simulink model "vehicle_model_2025"  (R2025a)
settings: Solver=ode23tb  StartTime=0.0  StopTime=20  MaxStep=0.001  RelTol=1e-3
model workspace (MAT data in the model file):
  init_r = 0
  init_vx = 0
  init_vy = 0
values from neighbouring files (symbols this model uses):
  Par =     [0_Load_data.mat]
  TireData =     [0_Load_data.mat]
undefined symbols (not defined in the file or in its folder): aero_par, Battery, Motor, SimInput_Steer, SimInput_TorqueFL, SimInput_TorqueFR, SimInput_TorqueRL, SimInput_TorqueRR, sus_par
libraries: simulink x4, BatteryEstimators x1
(part 1 of 2)
settings Model: PauseTimes=0  PacingRate=0.001000  Creator=rajde  LastModifiedBy=vishal bhujbal
settings DataIOCC: SaveOutput=off  SaveTime=off
settings DebuggingCC: UnderSpecifiedDimensionMsg=warning

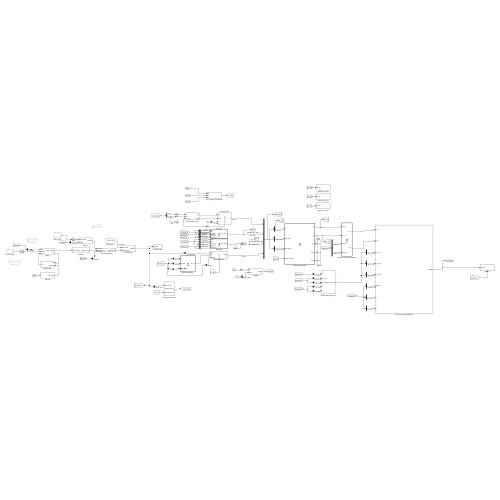
[thumbnail: Simulink's stored preview of the top-level diagram]
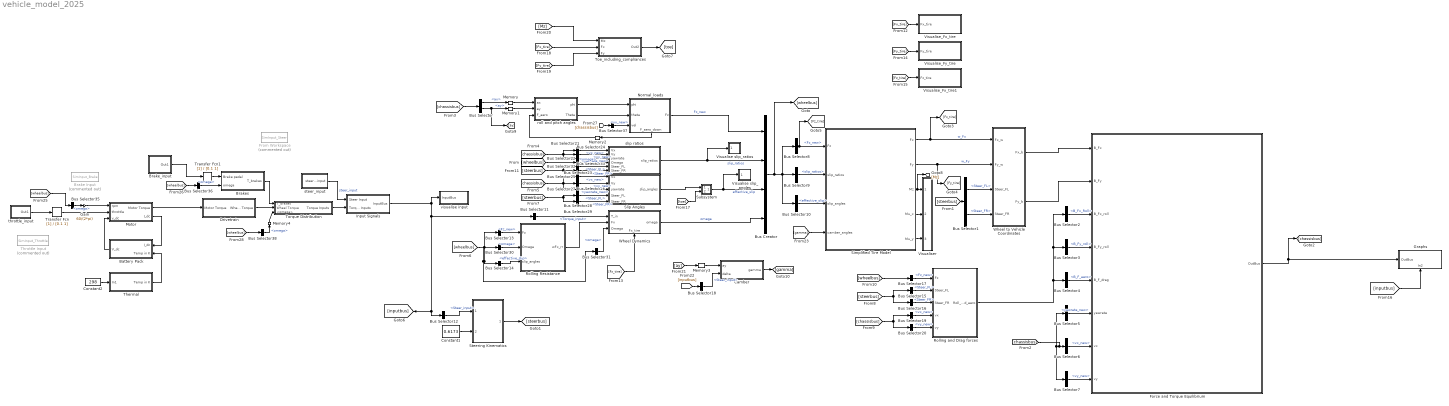
== system vehicle_model_2025 ==
  Battery Pack : Subsystem
  Brake Input : FromWorkspace  Commented=on  VariableName=SimInput_Brake
  Brake_input : Subsystem
  Brakes : Subsystem
  Bus Creator : BusCreator  Inputs=4
  Bus Selector : BusSelector  OutputSignals=ax,ay
  Bus Selector1 : BusSelector  OutputSignals=Steer_FL,Steer_FR
  Bus Selector10 : BusSelector  OutputSignals=effective_slip
  Bus Selector11 : BusSelector  OutputSignals=Torque_input
  Bus Selector12 : BusSelector  OutputSignals=Steer_input
  Bus Selector13 : BusSelector  OutputSignals=Fz_new
  Bus Selector14 : BusSelector  OutputSignals=effective_slip
  Bus Selector15 : BusSelector  OutputSignals=Steer_FL
  Bus Selector16 : BusSelector  OutputSignals=Steer_FR
  Bus Selector17 : BusSelector  OutputSignals=Fz_new
  Bus Selector18 : BusSelector  OutputSignals=Steer_input
  Bus Selector{6,19,21,25,37} (5 alike) : BusSelector  OutputSignals=vx_new
  Bus Selector2 : BusSelector  OutputSignals=B_Fx_Roll
  Bus Selector{7,20,24,26} (4 alike) : BusSelector  OutputSignals=vy_new
  Bus Selector22 : BusSelector  OutputSignals=yawrate_new
  Bus Selector{23,30..31,35..36,38} (6 alike) : BusSelector  OutputSignals=omega
  Bus Selector27 : BusSelector  OutputSignals=yawrate_new
  Bus Selector28 : BusSelector  OutputSignals=Steer_FL
  Bus Selector29 : BusSelector  OutputSignals=Steer_FR
  Bus Selector3 : BusSelector  OutputSignals=B_Fy_roll
  Bus Selector32 : BusSelector  OutputSignals=Steer_FL
  Bus Selector33 : BusSelector  OutputSignals=Steer_FR
  Bus Selector4 : BusSelector  OutputSignals=B_F_aero
  Bus Selector5 : BusSelector  OutputSignals=yawrate_new
  Bus Selector8 : BusSelector  OutputSignals=Fz_new
  Bus Selector9 : BusSelector  OutputSignals=slip_ratios
  Camber : Subsystem
  Constant1 : Constant  Value=0.6173
  Constant2 : Constant  Value=298
  Drivetrain : Subsystem
  Force and Torque Equilibrium : Subsystem
  From Workspace : FromWorkspace  Commented=on  VariableName=SimInput_Steer
  Gain : Gain  Gain=60/(2*pi)
  Graphs : Subsystem
      settings: PortSchema="{\"entries\":[{\"content\":{\"sides\":[{\"content\":{\"connectorIds\":[\"In1\"]},\"type\":\"ConnectorPlacement.EquallySpacedRectSide\",\"uuid\":\"0d7f1a6c-503e-4c9f-90e9-70f717dd7dfc\"},{\"content\":{\"side\":\"RIGHT\"},\"type\":\"ConnectorPlacement.EquallySpacedRectSide\",\"uuid\":\"62097468-b066-4e29-8f99-7427d14bee77\"},{\"content\":{\"side\":\"TOP\"},\"type\":\"ConnectorPlacement.EquallySpacedRectSide\",\"uuid\":\"2a3f381e-a201-4804-99b7-77b73504b102\"},{\"content\":{\"connectorIds\":[\"In2\"],\"side\":\"BOTTOM\"},\"type\":\"ConnectorPlacement.EquallySpacedRectSide\",\"uuid\":\"dae5de0a-879c-4844-a347-7056417d054f\"}]},\"type\":\"ConnectorPlacement.EquallySpacedConnector\",\"uuid\":\"aa2835d0-6748-4566-adf9-84e8214dd5a8\"}],\"packageUris\":[\"http://schema.mathworks.com/mf0/Connector/R2020b\"],\"version\":\"1.0\"}"
  Input Signals : Subsystem
  Memory : Memory  InheritSampleTime=on
  Memory1 : Memory  InheritSampleTime=on
  Memory2 : Memory  InheritSampleTime=on
  Memory3 : Memory
  Memory4 : Memory
  Motor : Subsystem
  Normal_loads : Subsystem
      settings: PortSchema="{\"entries\":[{\"content\":{\"sides\":[{\"content\":{\"connectorIds\":[\"In1\",\"In2\",\"In3\"]},\"type\":\"ConnectorPlacement.EquallySpacedRectSide\",\"uuid\":\"5b7db607-33bd-4d54-b958-3aa960e46147\"},{\"content\":{\"connectorIds\":[\"Out1\"],\"side\":\"RIGHT\"},\"type\":\"ConnectorPlacement.EquallySpacedRectSide\",\"uuid\":\"c12df481-c511-4c4c-afb1-8a5812ce44a5\"},{\"content\":{\"side\":\"TOP\"},\"type\":\"ConnectorPlacement.EquallySpacedRectSide\",\"uuid\":\"2c6024fe-fe45-4ba9-a61f-594b86562523\"},{\"content\":{\"connectorIds\":[\"Out2\"],\"side\":\"BOTTOM\"},\"type\":\"ConnectorPlacement.EquallySpacedRectSide\",\"uuid\":\"099189a9-186d-4ac0-a0af-1ec3a070ea03\"}]},\"type\":\"ConnectorPlacement.EquallySpacedConnector\",\"uuid\":\"81c2e338-68e5-401a-bb4f-0a973fbf41e6\"}],\"packageUris\":[\"http://schema.mathworks.com/mf0/Connector/R2020b\"],\"version\":\"1.0\"}"
  Rolling Resistance : MATLAB Function  TreatAsAtomicUnit=on
  Rolling and Drag forces : Subsystem
  Simplified Tire Model : MATLAB Function  TreatAsAtomicUnit=on
  Slip Angles : MATLAB Function  TreatAsAtomicUnit=on
  Steering Kinematics : Subsystem
  Subsystem : Subsystem
  Thermal : Subsystem
  Throttle Input : FromWorkspace  Commented=on  VariableName=SimInput_Throttle
  Toe_including_compliances : Subsystem
  Torque Distribution : Subsystem
  Transfer Fcn : TransferFcn  Denominator=[0.1 1]
  Transfer Fcn1 : TransferFcn  Denominator=[0.1 1]
  Visualise slip_angles : Subsystem
  Visualise slip_ratios : Subsystem
  Visualise_Fx_tire : Subsystem
  Visualise_Fx_tire1 : Subsystem
  Visualise_Fy_tire : Subsystem
  Visualiser : Subsystem
  Wheel Dynamics : Subsystem
      settings: PortSchema="{\"entries\":[{\"content\":{\"sides\":[{\"content\":{\"connectorIds\":[\"In1\",\"In2\",\"In3\"]},\"type\":\"ConnectorPlacement.EquallySpacedRectSide\",\"uuid\":\"f2e918e6-c6f6-4ec9-89f3-e2543a6374fd\"},{\"content\":{\"connectorIds\":[\"Out1\"],\"side\":\"RIGHT\"},\"type\":\"ConnectorPlacement.EquallySpacedRectSide\",\"uuid\":\"be700f5f-5cf3-4eec-a6f7-872bb7cd40f6\"},{\"content\":{\"side\":\"TOP\"},\"type\":\"ConnectorPlacement.EquallySpacedRectSide\",\"uuid\":\"c4f49273-9888-4d11-a98e-35dc6f585916\"},{\"content\":{\"connectorIds\":[\"In4\"],\"side\":\"BOTTOM\"},\"type\":\"ConnectorPlacement.EquallySpacedRectSide\",\"uuid\":\"8d2e7982-4362-4abb-b8fe-c155beeed1bc\"}]},\"type\":\"ConnectorPlacement.EquallySpacedConnector\",\"uuid\":\"4d6dafa1-905e-4e38-a48b-73a98e690073\"}],\"packageUris\":[\"http://schema.mathworks.com/mf0/Connector/R2020b\"],\"version\":\"1.0\"}"
  Wheel to Vehicle Coordinates : MATLAB Function  TreatAsAtomicUnit=on
  roll and pitch angles : Subsystem
  slip ratios : MATLAB Function  TreatAsAtomicUnit=on
  steer_input : Subsystem
  throttle_input : Subsystem
  visualise input : Subsystem
  wires:
  Simplified Tire Model/3(Mz) -> [Mz], Visualiser/1(mz)
  Simplified Tire Model/4(Mu_x) -> Visualiser/2(mu_x)
  Simplified Tire Model/5(Mu_y) -> Visualiser/3(mu_y)
  Simplified Tire Model/2(Fy) -> Wheel to Vehicle Coordinates/2(Fy_w), [Fy_tire]  "w_Fy"
  Simplified Tire Model/1(Fx) -> Wheel to Vehicle Coordinates/1(Fx_w), [Fx_tire]  "w_Fx"
  Wheel to Vehicle Coordinates/2(Fy_b) -> Force and Torque Equilibrium/2(B_Fy)
  Wheel to Vehicle Coordinates/1(Fx_b) -> Force and Torque Equilibrium/1(B_Fx)
  slip ratios/1(slip_ratios) -> Visualise slip_ratios/1(Kappa), Bus Creator/2  "slip_ratios"
  Wheel Dynamics/1(omega) -> Bus Creator/4  "omega"
  Bus Selector/1 -> Memory/1  "<ax>"
  Rolling Resistance/1(wFx_rr) -> Wheel Dynamics/2(Fx)
  Bus Selector1/1 -> Wheel to Vehicle Coordinates/3(Steer_FL)  "<Steer_FL>"
  Bus Selector1/2 -> Wheel to Vehicle Coordinates/4(Steer_FR)  "<Steer_FR>"
  Rolling and Drag forces/1(Roll_and_aero) -> Bus Selector2/1, Bus Selector3/1, Bus Selector4/1
  Bus Selector2/1 -> Force and Torque Equilibrium/3(B_Fx_roll)  "<B_Fx_Roll>"
  Bus Selector3/1 -> Force and Torque Equilibrium/4(B_Fy_roll)  "<B_Fy_roll>"
  Bus Selector4/1 -> Force and Torque Equilibrium/5(B_F_drag)  "<B_F_aero>"
  Bus Selector5/1 -> Force and Torque Equilibrium/6(yawrate)  "<yawrate_new>"
  Force and Torque Equilibrium/1(OutBus) -> [chassisbus], Graphs/1(OutBus)
  Bus Selector7/1 -> Force and Torque Equilibrium/8(vy)  "<vy_new>"
  Bus Selector6/1 -> Force and Torque Equilibrium/7(vx)  "<vx_new>"
  Bus Selector8/1 -> [Fz_tire], Simplified Tire Model/1(Fz)  "<Fz_new>"
  Bus Selector10/1 -> Simplified Tire Model/3(slip_angles)  "<effective_slip>"
  Bus Selector9/1 -> Simplified Tire Model/2(slip_ratios)  "<slip_ratios>"
  Bus Creator/1 -> [wheelbus], Bus Selector10/1, Bus Selector8/1, Bus Selector9/1
  Bus Selector12/1 -> Steering Kinematics/1(Steer_Input)  "<Steer_input>"
  Bus Selector11/1 -> Wheel Dynamics/1(T_in)  "<Torque_input>"
  Input Signals/1(InputBus) -> visualise input/1(InputBus), Bus Selector12/1, [inputbus], Bus Selector11/1
  Bus Selector14/1 -> Rolling Resistance/3(slip_angles)  "<effective_slip>"
  Bus Selector15/1 -> Rolling and Drag forces/2(Steer_FL)  "<Steer_FL>"
  Bus Selector16/1 -> Rolling and Drag forces/3(Steer_FR)  "<Steer_FR>"
  Constant1/1 -> Steering Kinematics/2(Ackermann_Pct)
  Bus Selector17/1 -> Rolling and Drag forces/1(Fz)  "<Fz_new>"
  Bus Selector19/1 -> Rolling and Drag forces/4(vx)  "<vx_new>"
  Bus Selector20/1 -> Rolling and Drag forces/5(vy)  "<vy_new>"
  Bus Selector21/1 -> slip ratios/1(Vx)  "<vx_new>"
  Bus Selector22/1 -> slip ratios/3(yawrate)  "<yawrate_new>"
  Bus Selector23/1 -> slip ratios/4(Omega)  "<omega>"
  Bus Selector25/1 -> Slip Angles/1(Vx)  "<vx_new>"
  Bus Selector26/1 -> Slip Angles/2(Vy)  "<vy_new>"
  Bus Selector27/1 -> Slip Angles/3(yawrate)  "<yawrate_new>"
  Bus Selector28/1 -> Slip Angles/4(Steer_FL)  "<Steer_FL>"
  Bus Selector29/1 -> Slip Angles/5(Steer_FR)  "<Steer_FR>"
  Steering Kinematics/1(Steering Angles) -> [steerbus]
  [steerbus] -> Bus Selector1/1
  [chassisbus] -> Bus Selector5/1, Bus Selector7/1, Bus Selector6/1
  [chassisbus] -> Bus Selector/1
  Bus Selector/2 -> Memory1/1, [ay]  "<ay>"
  [wheelbus] -> Bus Selector23/1
  [chassisbus] -> Bus Selector22/1, Bus Selector24/1, Bus Selector21/1
  [chassisbus] -> Bus Selector27/1, Bus Selector26/1, Bus Selector25/1
  [steerbus] -> Bus Selector29/1, Bus Selector28/1
  [wheelbus] -> Bus Selector13/1, Bus Selector30/1, Bus Selector14/1, Bus Selector31/1
  Bus Selector30/1 -> Rolling Resistance/2(Omega)  "<omega>"
  Bus Selector31/1 -> Wheel Dynamics/3(Omega)  "<omega>"
  [steerbus] -> Bus Selector16/1, Bus Selector15/1
  [chassisbus] -> Bus Selector20/1, Bus Selector19/1
  [wheelbus] -> Bus Selector17/1
  Bus Selector24/1 -> slip ratios/2(Vy)  "<vy_new>"
  Bus Selector33/1 -> slip ratios/6(Steer_FR)  "<Steer_FR>"
  [steerbus] -> Bus Selector32/1, Bus Selector33/1
  Bus Selector32/1 -> slip ratios/5(Steer_FL)  "<Steer_FL>"
  [Fx_tire] -> Wheel Dynamics/4(Fx_tire)
  Bus Selector13/1 -> Rolling Resistance/1(Fz)  "<Fz_new>"
  [inputbus] -> Graphs/2(In2)
  Slip Angles/1(slip_angles) -> Subsystem/1(slip_angles)
  [toe] -> Subsystem/2(toe)
  Subsystem/1(Out1) -> Visualise slip_angles/1(slip_angles), Bus Creator/3  "effective_slip"
  [Mz] -> Toe_including_compliances/1(Mz)
  [Fx_tire] -> Toe_including_compliances/2(Fx)
  [Fy_tire] -> Toe_including_compliances/3(Fy)
  Toe_including_compliances/1(Out2) -> [toe]
  [ay] -> Memory3/1
  [inputbus] -> Bus Selector18/1
  Bus Selector18/1 -> Camber/2(delta)  "<Steer_input>"
  Camber/1(gamma) -> [gamma]
  [gamma] -> Simplified Tire Model/4(camber_angles)
  roll and pitch angles/2(Theta) -> Normal_loads/2(theta)
  Memory/1 -> roll and pitch angles/1(ax)
  Memory1/1 -> roll and pitch angles/2(ay)
  Memory3/1 -> Camber/1(ay)
  Memory2/1 -> roll and pitch angles/3(F_aero)
  Brakes/1(T_brakes) -> Torque Distribution/1(T_brakes)
  Motor/1(Motor Torque) -> Drivetrain/1(Motor Torque)
  Bus Selector38/1 -> Memory4/1  "<omega>"
  Bus Selector35/1 -> Gain/1  "<omega>"
  Transfer Fcn/1 -> Motor/2(throttle)
  [wheelbus] -> Bus Selector36/1
  Brake_input/1(Out1) -> Transfer Fcn1/1
  Transfer Fcn1/1 -> Brakes/1(Brake pedal)
  Drivetrain/1(Wheel Torque) -> Torque Distribution/2(Wheel Torque)
  Thermal/1(Temp in K) -> Battery Pack/2(Temp in K)
  Constant2/1 -> Thermal/1(In1)
  Gain/1 -> Motor/1(rpm)
  [wheelbus] -> Bus Selector35/1
  Motor/2(I_dc) -> Battery Pack/1(I_dc)
  Bus Selector36/1 -> Brakes/2(omega)  "<omega>"
  throttle_input/1(Out1) -> Transfer Fcn/1
  Torque Distribution/1(Torque Inputs) -> Input Signals/2(Torque Inputs)
  Battery Pack/1(V_dc) -> Motor/3(v_dc)
  [wheelbus] -> Bus Selector38/1
  steer_input/1(steer_input) -> Input Signals/1(Steer Input)  "steer_input"
  Memory4/1 -> Torque Distribution/3(<omega>)
  [Fy_tire] -> Visualise_Fy_tire/1(Fy_tire)
  [Fx_tire] -> Visualise_Fx_tire/1(Fx_tire)
  [Fz_tire] -> Visualise_Fx_tire1/1(Fz_tire)
  roll and pitch angles/1(phi) -> Normal_loads/1(phi)
  [chassisbus] -> Bus Selector37/1
  Bus Selector37/1 -> Normal_loads/3(vel)  "<vx_new>"
  Normal_loads/2(F_aero_down) -> Memory2/1
  Normal_loads/1(Fz) -> Bus Creator/1  "Fz_new"

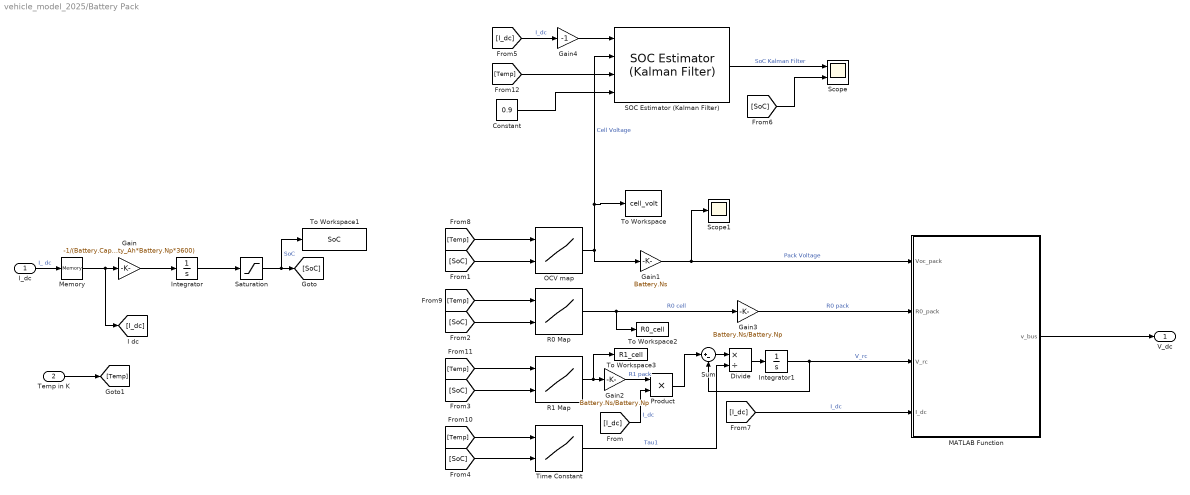
== system vehicle_model_2025/Battery Pack ==
  I_dc : Inport
  Temp in K : Inport  Port=2
  Constant : Constant  Value=0.9
  Divide : Product  Inputs=*/
  Gain : Gain  Gain=-1/(Battery.Capacity_Ah*Battery.Np*3600)
  Gain1 : Gain  Gain=Battery.Ns
  Gain2 : Gain  Gain=Battery.Ns/Battery.Np
  Gain3 : Gain  Gain=Battery.Ns/Battery.Np
  Gain4 : Gain  Gain=-1
  Integrator : Integrator  InitialCondition=1
  Integrator1 : Integrator
  MATLAB Function : MATLAB Function  TreatAsAtomicUnit=on
  Memory : Memory
  OCV map : Lookup_n-D  BreakpointsForDimension1=Battery.T_vec  BreakpointsForDimension2=Battery.SoC_vec  Table=Battery.OCV_map'  InternalRulePriority=Speed  RndMeth=Simplest
      settings: InputPortMap=u0,u1
  Product : Product
  R0 Map : Lookup_n-D  BreakpointsForDimension1=Battery.T_vec  BreakpointsForDimension2=Battery.SoC_vec  Table=Battery.R0_map'  InternalRulePriority=Speed  RndMeth=Simplest
      settings: InputPortMap=u0,u1
  R1 Map : Lookup_n-D  BreakpointsForDimension1=Battery.T_vec  BreakpointsForDimension2=Battery.SoC_vec  Table=Battery.R1_map'  InternalRulePriority=Speed  RndMeth=Simplest
      settings: InputPortMap=u0,u1
  SOC Estimator (Kalman Filter) : BatteryEstimators/SOC Estimator (Kalman Filter)  CurrentInputPartition=off  filterType=Extended Kalman filter  alpha=1  beta=2  kappa=0  Q=|  Q_2RC=|  R=0.1  P0=[1e-5 0; 0 1]  P0_2RC=[1e-5 0 0; 0 1 0;0 0 1]  Ts=1  chargeDynamics=One time-constant dynamics  SOC_vec=[0 0.1 0.25 0.5 0.75 0.9 1]  T_vec=[278 293 313]  R0_mat=[0.0117 0.0085 0.009;0.011 0.0085 0.009;0.0114 0.0087 0.0092;0.0107 0.0082 0.0088;0.0107 0.0083 0.0091;0.0113 0.0085 0.0089;0.0116 0.0085 0.0089]  R1_mat=[0.0109 0.0029 0.0013;0.0069 0.0024 0.0012;0.0047 0.0026 0.0013;0.0034 0.0016 0.001;0.0033 0.0023 0.0014;0.0033 0.0018 0.0011;0.0028 0.0017 0.0011]  tau1_mat=[20 36 39;31 45 39;109 105 61;36 29 26;59 77 67;40 33 29;25 39 33]  R2_mat=[.0109, .0029, .0013; .0069, .0024, .0012; .0047, .0026, .0013; .0034, .0016, .001; .0033, .0023, .0014; .0033, .0018, .0011; .0028, .0017, .0011]  tau2_mat=[20, 36, 39; 31, 45, 39; 109, 105, 61; 36, 29, 26; 59, 77, 67; 40, 33, 29; 25, 39, 33]  V0_mat=[3.49 3.5 3.51;3.55 3.57 3.56;3.62 3.63 3.64;3.71 3.71 3.72;3.91 3.93 3.94;4.07 4.08 4.08;4.19 4.19 4.19]  AH=4.493  DataType=Inherit: auto
      Q=|
      | [1e-6 0;
      | 0 1e-6]
      Q_2RC=|
      | [1e-6 0 0;
      | 0 1e-6 0; 0 0 1e-6]
      settings: LibrarySourceBlock=|
      | batt_sl_lib/Estimators/SOC Estimator
      | (Kalman Filter)
  Saturation : Saturate  UpperLimit=1  LowerLimit=0
  Scope : Scope  NumInputPorts=2
      settings: ActiveDisplayYMinimum=0.74077842215921907  ActiveDisplayYMaximum=0.86213619236438077  DataLoggingVariableName=ScopeData8
  Scope1 : Scope
      settings: ActiveDisplayYMinimum=583.02637249372378  ActiveDisplayYMaximum=588.01929194514184  DataLoggingVariableName=ScopeData14
  Sum : Sum  Inputs=|+-
  Time Constant : Lookup_n-D  BreakpointsForDimension1=Battery.T_vec  BreakpointsForDimension2=Battery.SoC_vec  Table=Battery.Tau_map'  InternalRulePriority=Speed  RndMeth=Simplest
      settings: InputPortMap=u0,u1
  To Workspace : ToWorkspace  VariableName=cell_volt  SaveFormat=Timeseries  SampleTime=-1
  To Workspace1 : ToWorkspace  VariableName=SoC  SaveFormat=Timeseries  SampleTime=-1
  To Workspace2 : ToWorkspace  VariableName=R0_cell  SaveFormat=Timeseries  SampleTime=-1
  To Workspace3 : ToWorkspace  VariableName=R1_cell  SaveFormat=Timeseries  SampleTime=-1
  V_dc : Outport
  wires:
  I_dc/1 -> Memory/1  "I_ dc"
  Gain/1 -> Integrator/1
  Integrator/1 -> Saturation/1
  OCV map/1 -> To Workspace/1, SOC Estimator (Kalman Filter)/2, Gain1/1  "Cell Voltage"
  Gain1/1 -> Scope1/1, MATLAB Function/1(Voc_pack)  "Pack Voltage"
  R1 Map/1 -> To Workspace3/1, Gain2/1
  R0 Map/1 -> To Workspace2/1, Gain3/1  "R0 cell"
  Gain3/1 -> MATLAB Function/2(R0_pack)  "R0 pack"
  Gain2/1 -> Product/1  "R1 pack"
  Product/1 -> Sum/1
  Integrator1/1 -> MATLAB Function/3(V_rc), Sum/2  "V_rc"
  Sum/1 -> Divide/1
  Time Constant/1 -> Divide/2  "Tau1"
  Divide/1 -> Integrator1/1
  Constant/1 -> SOC Estimator (Kalman Filter)/4
  SOC Estimator (Kalman Filter)/1 -> Scope/1  "SoC Kalman Filter"
  MATLAB Function/1(v_bus) -> V_dc/1
  [I_dc] -> Product/2  "I_dc"
  Saturation/1 -> To Workspace1/1, [SoC]  "SoC"
  [SoC] -> Time Constant/2
  [SoC] -> R1 Map/2
  [SoC] -> R0 Map/2
  [SoC] -> OCV map/2
  [I_dc] -> Gain4/1  "I_dc"
  [SoC] -> Scope/2
  [I_dc] -> MATLAB Function/4(I_dc)  "I_dc"
  Temp in K/1 -> [Temp]
  [Temp] -> OCV map/1
  [Temp] -> R0 Map/1
  [Temp] -> R1 Map/1
  [Temp] -> Time Constant/1
  [Temp] -> SOC Estimator (Kalman Filter)/3
  Memory/1 -> [I_dc], Gain/1
  Gain4/1 -> SOC Estimator (Kalman Filter)/1

== system vehicle_model_2025/Brake_input ==
  Constant4 : Constant  Value=0
  Out1 : Outport
  wires:
  Constant4/1 -> Out1/1

== system vehicle_model_2025/Brakes ==
  Brake pedal : Inport
  omega : Inport  Port=2
  MATLAB Function : MATLAB Function  TreatAsAtomicUnit=on
  T_brakes : Outport
  wires:
  MATLAB Function/1(T_brakes) -> T_brakes/1
  omega/1 -> MATLAB Function/2(omega)
  Brake pedal/1 -> MATLAB Function/1(brake_pedal)

== system vehicle_model_2025/Camber ==
  ay : Inport
  delta : Inport  Port=2
  MATLAB Function : MATLAB Function  TreatAsAtomicUnit=on
  Mux : Mux
  gamma : Outport
  wires:
  MATLAB Function/1(gamma_FR) -> Mux/1
  MATLAB Function/2(gamma_FL) -> Mux/2
  MATLAB Function/3(gamma_RL) -> Mux/3
  MATLAB Function/4(gamma_RR) -> Mux/4
  Mux/1 -> gamma/1
  ay/1 -> MATLAB Function/1(ay)
  delta/1 -> MATLAB Function/2(delta)

== system vehicle_model_2025/Drivetrain ==
  Motor Torque : Inport
  Gear Ratio : Gain  Gain=10.05
  Overall Powertrain Efficiency : Gain  Gain=0.83
  Wheel Torque : Outport
  wires:
  Motor Torque/1 -> Gear Ratio/1
  Gear Ratio/1 -> Overall Powertrain Efficiency/1
  Overall Powertrain Efficiency/1 -> Wheel Torque/1

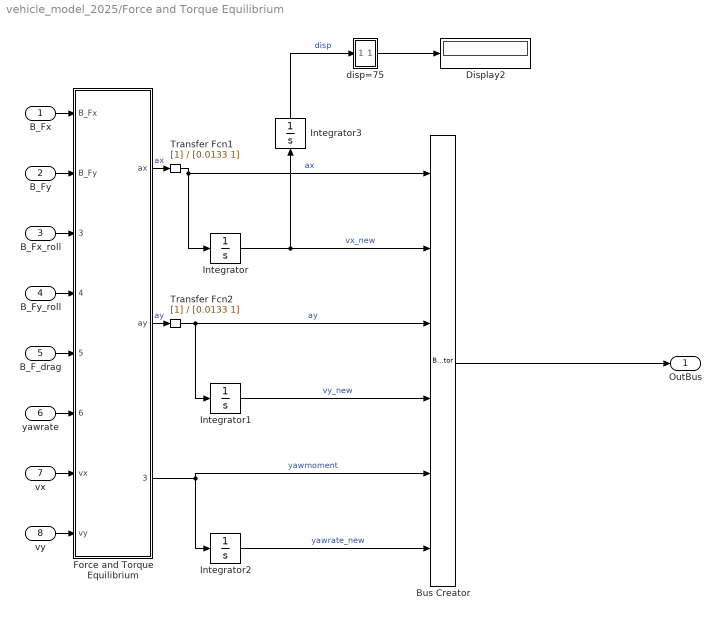
== system vehicle_model_2025/Force and Torque Equilibrium ==
  B_Fx : Inport
  B_Fy : Inport  Port=2
  B_Fx_roll : Inport  Port=3
  B_Fy_roll : Inport  Port=4
  B_F_drag : Inport  Port=5
  yawrate : Inport  Port=6
  vx : Inport  Port=7
  vy : Inport  Port=8
  Bus Creator : BusCreator  Inputs=6
  Display2 : Display
  Force and Torque Equilibrium : MATLAB Function  TreatAsAtomicUnit=on
  Integrator : Integrator  InitialCondition=init_vx  LimitOutput=on  UpperSaturationLimit=1e6  LowerSaturationLimit=0
  Integrator1 : Integrator  InitialCondition=init_vy  LimitOutput=on  UpperSaturationLimit=1e6
  Integrator2 : Integrator  InitialCondition=init_r  LimitOutput=on  UpperSaturationLimit=1e6
  Integrator3 : Integrator
  Transfer Fcn1 : TransferFcn  Denominator=[0.0133 1]
  Transfer Fcn2 : TransferFcn  Denominator=[0.0133 1]
  disp=75 : Subsystem
  OutBus : Outport
  wires:
  vy/1 -> Force and Torque Equilibrium/8(vy)
  B_Fx/1 -> Force and Torque Equilibrium/1(B_Fx)
  B_Fx_roll/1 -> Force and Torque Equilibrium/3(B_Fx_roll)
  B_F_drag/1 -> Force and Torque Equilibrium/5(B_F_drag)
  B_Fy/1 -> Force and Torque Equilibrium/2(B_Fy)
  B_Fy_roll/1 -> Force and Torque Equilibrium/4(B_Fy_roll)
  vx/1 -> Force and Torque Equilibrium/7(vx)
  Force and Torque Equilibrium/2(ay) -> Transfer Fcn2/1  "ay"
  Force and Torque Equilibrium/1(ax) -> Transfer Fcn1/1  "ax"
  Force and Torque Equilibrium/3(yawmoment) -> Integrator2/1, Bus Creator/5  "yawmoment"
  Integrator/1 -> Integrator3/1, Bus Creator/2  "vx_new"
  Integrator1/1 -> Bus Creator/4  "vy_new"
  Integrator2/1 -> Bus Creator/6  "yawrate_new"
  Bus Creator/1 -> OutBus/1
  yawrate/1 -> Force and Torque Equilibrium/6(yawrate)
  Transfer Fcn1/1 -> Integrator/1, Bus Creator/1  "ax"
  Transfer Fcn2/1 -> Integrator1/1, Bus Creator/3  "ay"
  disp=75/1(Out1) -> Display2/1
  Integrator3/1 -> disp=75/1(disp)  "disp"

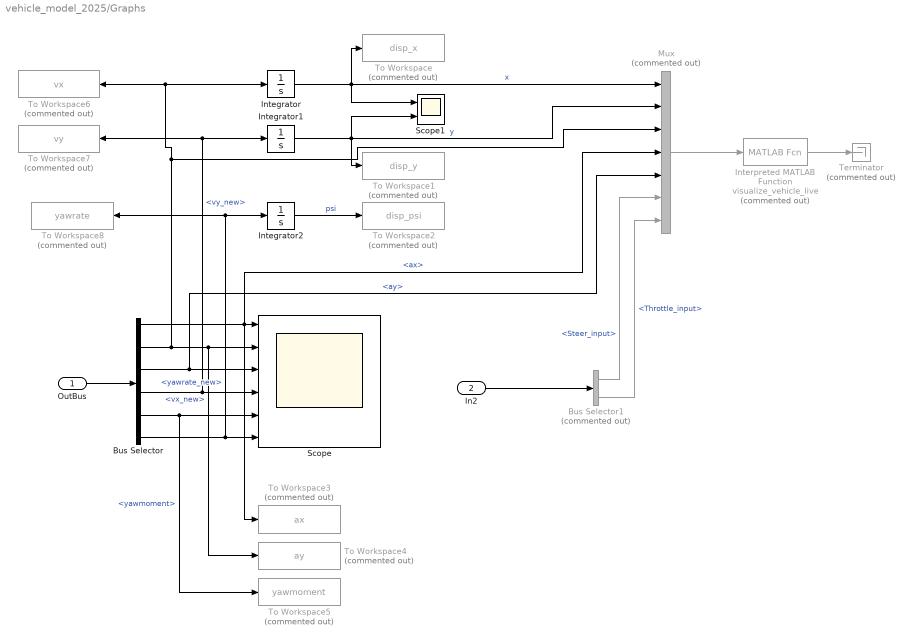
== system vehicle_model_2025/Graphs ==
  OutBus : Inport
  In2 : Inport  Port=2
  Bus Selector : BusSelector  OutputSignals=ax,vx_new,ay,vy_new,yawmoment,yawrate_new
  Bus Selector1 : BusSelector  Commented=on  OutputSignals=Steer_input,Throttle_input
  Integrator : Integrator
  Integrator1 : Integrator
  Integrator2 : Integrator
  Interpreted MATLAB Function : MATLABFcn  Commented=on  MATLABFcn=visualize_vehicle_live
  Mux : Mux  Commented=on  Inputs=7
  Scope : Scope  NumInputPorts=6
      settings: ActiveDisplayYMinimum=-0.80061135979916376  ActiveDisplayYMaximum=6.9634265458567022  DataLoggingVariableName=ScopeData2
  Scope1 : Scope  NumInputPorts=2
      settings: ActiveDisplayYMinimum=-673.27901203322881  ActiveDisplayYMaximum=6059.5111082990607  DataLoggingVariableName=ScopeData7
  Terminator : Terminator  Commented=on
  To Workspace : ToWorkspace  Commented=on  VariableName=disp_x  SaveFormat=Timeseries  SampleTime=-1
  To Workspace1 : ToWorkspace  Commented=on  VariableName=disp_y  SaveFormat=Timeseries  SampleTime=-1
  To Workspace2 : ToWorkspace  Commented=on  VariableName=disp_psi  SaveFormat=Timeseries  SampleTime=-1
  To Workspace3 : ToWorkspace  Commented=on  VariableName=ax  SaveFormat=Timeseries  SampleTime=-1
  To Workspace4 : ToWorkspace  Commented=on  VariableName=ay  SaveFormat=Timeseries  SampleTime=-1
  To Workspace5 : ToWorkspace  Commented=on  VariableName=yawmoment  SaveFormat=Timeseries  SampleTime=-1
  To Workspace6 : ToWorkspace  Commented=on  VariableName=vx  SaveFormat=Timeseries  SampleTime=-1
  To Workspace7 : ToWorkspace  Commented=on  VariableName=vy  SaveFormat=Timeseries  SampleTime=-1
  To Workspace8 : ToWorkspace  Commented=on  VariableName=yawrate  SaveFormat=Timeseries  SampleTime=-1
  wires:
  OutBus/1 -> Bus Selector/1
  Bus Selector/1 -> To Workspace3/1, Scope/1, Mux/4  "<ax>"
  Bus Selector/2 -> To Workspace6/1, Integrator/1, Mux/3, To Workspace4/1, Scope/2  "<vx_new>"
  Bus Selector/3 -> Mux/5, Scope/3  "<ay>"
  Bus Selector/4 -> To Workspace7/1, Integrator1/1, Scope/4  "<vy_new>"
  Bus Selector/5 -> To Workspace5/1, Scope/5  "<yawmoment>"
  Bus Selector/6 -> To Workspace8/1, Integrator2/1, Scope/6  "<yawrate_new>"
  Integrator/1 -> Scope1/1, Mux/1, To Workspace/1  "x"
  Integrator1/1 -> Scope1/2, Mux/2, To Workspace1/1  "y"
  Integrator2/1 -> To Workspace2/1  "psi"
  Mux/1 -> Interpreted MATLAB Function/1
  Interpreted MATLAB Function/1 -> Terminator/1
  In2/1 -> Bus Selector1/1
  Bus Selector1/1 -> Mux/6  "<Steer_input>"
  Bus Selector1/2 -> Mux/7  "<Throttle_input>"

== system vehicle_model_2025/Input Signals ==
  Steer Input : Inport
  Torque Inputs : Inport  Port=2
  Bus Creator : BusCreator  Inputs=2
  InputBus : Outport
  wires:
  Torque Inputs/1 -> Bus Creator/1  "Torque_input"
  Steer Input/1 -> Bus Creator/2  "Steer_input"
  Bus Creator/1 -> InputBus/1

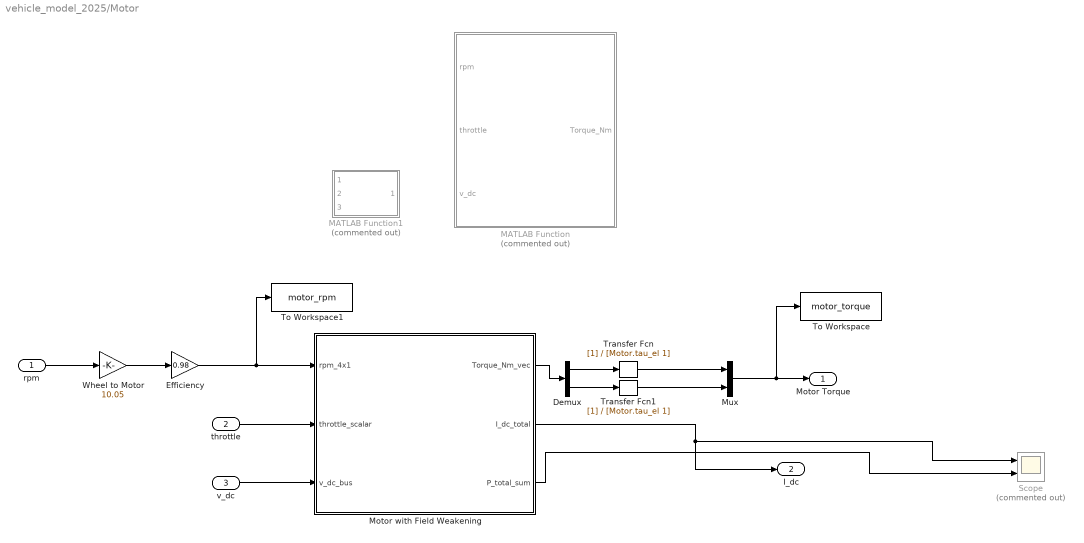
== system vehicle_model_2025/Motor ==
  rpm : Inport
  throttle : Inport  Port=2
  v_dc : Inport  Port=3
  Demux : Demux  Outputs=2
  Efficiency : Gain  Gain=0.98
  MATLAB Function : MATLAB Function  Commented=on  TreatAsAtomicUnit=on
  MATLAB Function1 : MATLAB Function  Commented=on  TreatAsAtomicUnit=on
  Motor with Field Weakening : MATLAB Function  TreatAsAtomicUnit=on
  Mux : Mux  Inputs=2
  Scope : Scope  Commented=on  NumInputPorts=2
      settings: ActiveDisplayYMinimum=-1  ActiveDisplayYMaximum=1  DataLoggingVariableName=ScopeData9
  To Workspace : ToWorkspace  VariableName=motor_torque  SaveFormat=Timeseries  SampleTime=-1
  To Workspace1 : ToWorkspace  VariableName=motor_rpm  SaveFormat=Timeseries  SampleTime=-1
  Transfer Fcn : TransferFcn  Denominator=[Motor.tau_el 1]
  Transfer Fcn1 : TransferFcn  Denominator=[Motor.tau_el 1]
  Wheel to Motor : Gain  Gain=10.05
  Motor Torque : Outport
  I_dc : Outport  Port=2
  wires:
  rpm/1 -> Wheel to Motor/1
  throttle/1 -> Motor with Field Weakening/2(throttle_scalar)
  v_dc/1 -> Motor with Field Weakening/3(v_dc_bus)
  Wheel to Motor/1 -> Efficiency/1
  Efficiency/1 -> To Workspace1/1, Motor with Field Weakening/1(rpm_4x1)
  Motor with Field Weakening/2(I_dc_total) -> I_dc/1, Scope/1
  Motor with Field Weakening/1(Torque_Nm_vec) -> Demux/1
  Demux/1 -> Transfer Fcn/1
  Transfer Fcn1/1 -> Mux/2
  Demux/2 -> Transfer Fcn1/1
  Transfer Fcn/1 -> Mux/1
  Mux/1 -> To Workspace/1, Motor Torque/1
  Motor with Field Weakening/3(P_total_sum) -> Scope/2

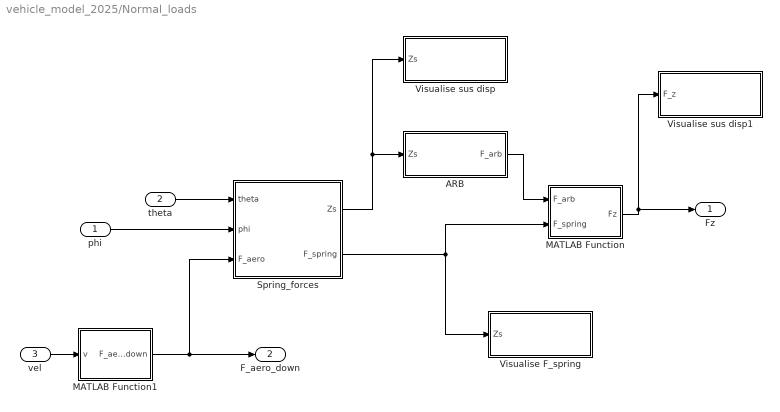
== system vehicle_model_2025/Normal_loads ==
  phi : Inport
  theta : Inport  Port=2
  vel : Inport  Port=3
  ARB : Subsystem
  MATLAB Function : MATLAB Function  TreatAsAtomicUnit=on
  MATLAB Function1 : MATLAB Function  TreatAsAtomicUnit=on
  Spring_forces : Subsystem
  Visualise F_spring : Subsystem
  Visualise sus disp : Subsystem
  Visualise sus disp1 : Subsystem
  Fz : Outport
  F_aero_down : Outport  Port=2
  wires:
  theta/1 -> Spring_forces/1(theta)
  phi/1 -> Spring_forces/2(phi)
  Spring_forces/1(Zs) -> Visualise sus disp/1(Zs), ARB/1(Zs)
  Spring_forces/2(F_spring) -> Visualise F_spring/1(Zs), MATLAB Function/2(F_spring)
  ARB/1(F_arb) -> MATLAB Function/1(F_arb)
  MATLAB Function/1(Fz) -> Visualise sus disp1/1(F_z), Fz/1
  vel/1 -> MATLAB Function1/1(v)
  MATLAB Function1/1(F_aero_down) -> Spring_forces/3(F_aero), F_aero_down/1

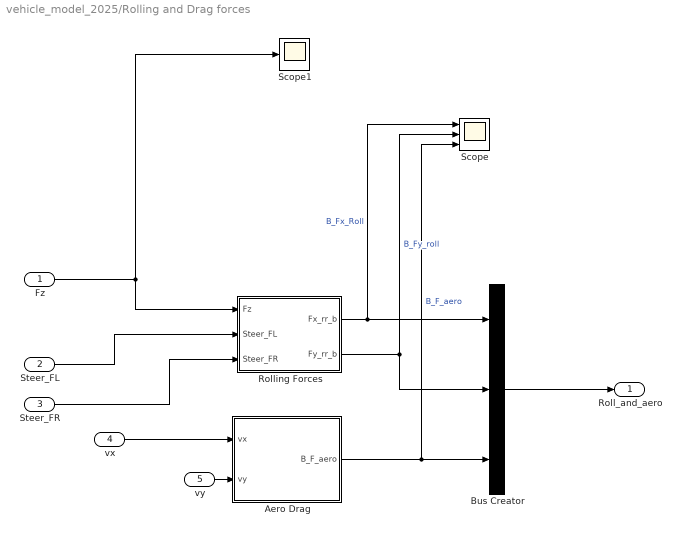
== system vehicle_model_2025/Rolling and Drag forces ==
  Fz : Inport
  Steer_FL : Inport  Port=2
  Steer_FR : Inport  Port=3
  vx : Inport  Port=4
  vy : Inport  Port=5
  Aero Drag : MATLAB Function  TreatAsAtomicUnit=on
  Bus Creator : BusCreator  Inputs=3
  Rolling Forces : MATLAB Function  TreatAsAtomicUnit=on
  Scope : Scope  NumInputPorts=3
      settings: ActiveDisplayYMinimum=-84.954759082659436  ActiveDisplayYMaximum=8.7114722532307756  DataLoggingVariableName=ScopeData5
  Scope1 : Scope
      settings: ActiveDisplayYMinimum=-1  ActiveDisplayYMaximum=1  DataLoggingVariableName=ScopeData6
  Roll_and_aero : Outport
  wires:
  Steer_FL/1 -> Rolling Forces/2(Steer_FL)
  vx/1 -> Aero Drag/1(vx)
  Fz/1 -> Scope1/1, Rolling Forces/1(Fz)
  Aero Drag/1(B_F_aero) -> Bus Creator/3, Scope/3  "B_F_aero"
  Rolling Forces/1(Fx_rr_b) -> Scope/1, Bus Creator/1  "B_Fx_Roll"
  Steer_FR/1 -> Rolling Forces/3(Steer_FR)
  vy/1 -> Aero Drag/2(vy)
  Rolling Forces/2(Fy_rr_b) -> Bus Creator/2, Scope/2  "B_Fy_roll"
  Bus Creator/1 -> Roll_and_aero/1

== system vehicle_model_2025/Steering Kinematics ==
  Steer_Input : Inport
  Ackermann_Pct : Inport  Port=2
  Bus Creator1 : BusCreator  Inputs=2
  Steering Kinematics : MATLAB Function  TreatAsAtomicUnit=on
  Steering Angles : Outport
  wires:
  Steering Kinematics/1(Steer_FL) -> Bus Creator1/1  "Steer_FL"
  Steer_Input/1 -> Steering Kinematics/1(Steer_Input)
  Steering Kinematics/2(Steer_FR) -> Bus Creator1/2  "Steer_FR"
  Ackermann_Pct/1 -> Steering Kinematics/2(Ackermann_Pct)
  Bus Creator1/1 -> Steering Angles/1

== system vehicle_model_2025/Subsystem ==
  slip_angles : Inport
  toe : Inport  Port=2
  Subtract : Sum  Inputs=+-
  Out1 : Outport
  wires:
  slip_angles/1 -> Subtract/1
  toe/1 -> Subtract/2
  Subtract/1 -> Out1/1

== system vehicle_model_2025/Thermal ==
  In1 : Inport
  Temp in K : Outport
  wires:
  In1/1 -> Temp in K/1

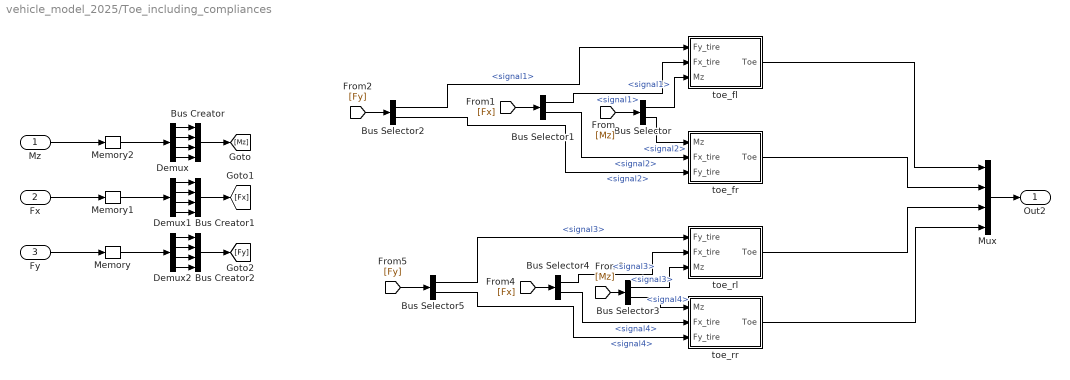
== system vehicle_model_2025/Toe_including_compliances ==
  Mz : Inport
  Fx : Inport  Port=2
  Fy : Inport  Port=3
  Bus Creator : BusCreator  Inputs=4
  Bus Creator1 : BusCreator  Inputs=4
  Bus Creator2 : BusCreator  Inputs=4
  Bus Selector : BusSelector  OutputSignals=signal1,signal2
  Bus Selector1 : BusSelector  OutputSignals=signal1,signal2
  Bus Selector2 : BusSelector  OutputSignals=signal1,signal2
  Bus Selector3 : BusSelector  OutputSignals=signal3,signal4
  Bus Selector4 : BusSelector  OutputSignals=signal3,signal4
  Bus Selector5 : BusSelector  OutputSignals=signal3,signal4
  Demux : Demux
  Demux1 : Demux
  Demux2 : Demux
  Memory : Memory
  Memory1 : Memory
  Memory2 : Memory
  Mux : Mux
  toe_fl : MATLAB Function  TreatAsAtomicUnit=on
  toe_fr : MATLAB Function  TreatAsAtomicUnit=on
  toe_rl : MATLAB Function  TreatAsAtomicUnit=on
  toe_rr : MATLAB Function  TreatAsAtomicUnit=on
  Out2 : Outport
  wires:
  Mz/1 -> Memory2/1
  Demux/1 -> Bus Creator/1
  Demux/2 -> Bus Creator/2
  Demux/3 -> Bus Creator/3
  Demux/4 -> Bus Creator/4
  Bus Creator/1 -> [Mz]
  [Mz] -> Bus Selector/1
  Bus Selector/1 -> toe_fl/3(Mz)  "<signal1>"
  Bus Selector/2 -> toe_fr/1(Mz)  "<signal2>"
  Fx/1 -> Memory1/1
  Demux1/1 -> Bus Creator1/1
  Demux1/2 -> Bus Creator1/2
  Demux1/3 -> Bus Creator1/3
  Demux1/4 -> Bus Creator1/4
  Bus Creator1/1 -> [Fx]
  Fy/1 -> Memory/1
  Demux2/1 -> Bus Creator2/1
  Demux2/2 -> Bus Creator2/2
  Demux2/3 -> Bus Creator2/3
  Demux2/4 -> Bus Creator2/4
  Bus Creator2/1 -> [Fy]
  [Fx] -> Bus Selector1/1
  Bus Selector1/1 -> toe_fl/2(Fx_tire)  "<signal1>"
  Bus Selector1/2 -> toe_fr/2(Fx_tire)  "<signal2>"
  [Fy] -> Bus Selector2/1
  Bus Selector2/1 -> toe_fl/1(Fy_tire)  "<signal1>"
  Bus Selector2/2 -> toe_fr/3(Fy_tire)  "<signal2>"
  Bus Selector3/1 -> toe_rl/3(Mz)  "<signal3>"
  [Mz] -> Bus Selector3/1
  [Fx] -> Bus Selector4/1
  [Fy] -> Bus Selector5/1
  Bus Selector3/2 -> toe_rr/1(Mz)  "<signal4>"
  Bus Selector4/1 -> toe_rl/2(Fx_tire)  "<signal3>"
  Bus Selector4/2 -> toe_rr/2(Fx_tire)  "<signal4>"
  Bus Selector5/1 -> toe_rl/1(Fy_tire)  "<signal3>"
  Bus Selector5/2 -> toe_rr/3(Fy_tire)  "<signal4>"
  toe_fl/1(Toe) -> Mux/1
  toe_fr/1(Toe) -> Mux/2
  toe_rl/1(Toe) -> Mux/3
  toe_rr/1(Toe) -> Mux/4
  Mux/1 -> Out2/1
  Memory/1 -> Demux2/1
  Memory1/1 -> Demux1/1
  Memory2/1 -> Demux/1

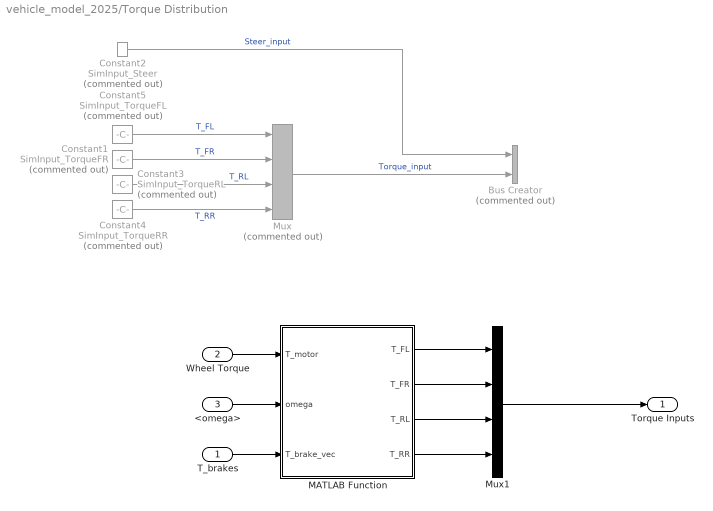
== system vehicle_model_2025/Torque Distribution ==
  T_brakes : Inport
  Wheel Torque : Inport  Port=2
  <omega> : Inport  Port=3
  Bus Creator : BusCreator  Commented=on  Inputs=2
  Constant1 : Constant  Commented=on  Value=SimInput_TorqueFR
  Constant2 : Constant  Commented=on  Value=SimInput_Steer
  Constant3 : Constant  Commented=on  Value=SimInput_TorqueRL
  Constant4 : Constant  Commented=on  Value=SimInput_TorqueRR
  Constant5 : Constant  Commented=on  Value=SimInput_TorqueFL
  MATLAB Function : MATLAB Function  TreatAsAtomicUnit=on
  Mux : Mux  Commented=on
  Mux1 : Mux
  Torque Inputs : Outport
  wires:
  Mux/1 -> Bus Creator/2  "Torque_input"
  Constant2/1 -> Bus Creator/1  "Steer_input"
  Constant4/1 -> Mux/4  "T_RR"
  Constant1/1 -> Mux/2  "T_FR"
  Constant3/1 -> Mux/3  "T_RL"
  Constant5/1 -> Mux/1  "T_FL"
  Wheel Torque/1 -> MATLAB Function/1(T_motor)
  T_brakes/1 -> MATLAB Function/3(T_brake_vec)
  MATLAB Function/1(T_FL) -> Mux1/1
  MATLAB Function/2(T_FR) -> Mux1/2
  MATLAB Function/3(T_RL) -> Mux1/3
  MATLAB Function/4(T_RR) -> Mux1/4
  Mux1/1 -> Torque Inputs/1
  <omega>/1 -> MATLAB Function/2(omega)

== system vehicle_model_2025/Visualise slip_angles ==
  slip_angles : Inport
  MATLAB Function : MATLAB Function  TreatAsAtomicUnit=on
  To Workspace : ToWorkspace  VariableName=slip_angle_fl  SaveFormat=Timeseries  SampleTime=-1
  To Workspace1 : ToWorkspace  VariableName=slip_angle_fr  SaveFormat=Timeseries  SampleTime=-1
  To Workspace2 : ToWorkspace  VariableName=slip_angle_rl  SaveFormat=Timeseries  SampleTime=-1
  To Workspace3 : ToWorkspace  VariableName=slip_angle_rr  SaveFormat=Timeseries  SampleTime=-1
  Visualise slip_angle : Scope  NumInputPorts=4
      settings: ActiveDisplayYMinimum=-1  ActiveDisplayYMaximum=1  DataLoggingVariableName=ScopeData3
  wires:
  MATLAB Function/4(alpha_rr) -> To Workspace3/1, Visualise slip_angle/4  "alpha_rr"
  MATLAB Function/3(alpha_rl) -> To Workspace2/1, Visualise slip_angle/3  "alpha_rl"
  MATLAB Function/2(alpha_fr) -> To Workspace1/1, Visualise slip_angle/2  "alpha_fr"
  MATLAB Function/1(alpha_fl) -> To Workspace/1, Visualise slip_angle/1  "alpha_fl"
  slip_angles/1 -> MATLAB Function/1(slip_angles)

== system vehicle_model_2025/Visualise slip_ratios ==
  Kappa : Inport
  MATLAB Function : MATLAB Function  TreatAsAtomicUnit=on
  To Workspace : ToWorkspace  VariableName=slip_ratio_fl  SaveFormat=Timeseries  SampleTime=-1
  To Workspace1 : ToWorkspace  VariableName=slip_ratio_fr  SaveFormat=Timeseries  SampleTime=-1
  To Workspace2 : ToWorkspace  VariableName=slip_ratio_rl  SaveFormat=Timeseries  SampleTime=-1
  To Workspace3 : ToWorkspace  VariableName=slip_ratio_rr  SaveFormat=Timeseries  SampleTime=-1
  Visualise slip_ratio : Scope  NumInputPorts=4
      settings: ActiveDisplayYMinimum=-1  ActiveDisplayYMaximum=1  DataLoggingVariableName=ScopeData3
  wires:
  Kappa/1 -> MATLAB Function/1(kappa)
  MATLAB Function/1(K_fl) -> Visualise slip_ratio/1, To Workspace/1  "slip_ratio_fl"
  MATLAB Function/2(K_fr) -> Visualise slip_ratio/2, To Workspace1/1  "slip_ratio_fr"
  MATLAB Function/3(K_rl) -> Visualise slip_ratio/3, To Workspace2/1  "slip_ratio_rl"
  MATLAB Function/4(K_rr) -> Visualise slip_ratio/4, To Workspace3/1  "slip_ratio_rr"

== system vehicle_model_2025/Visualise_Fx_tire ==
  Fx_tire : Inport
  MATLAB Function : MATLAB Function  TreatAsAtomicUnit=on
  To Workspace : ToWorkspace  VariableName=Fx_fl  SaveFormat=Timeseries  SampleTime=-1
  To Workspace1 : ToWorkspace  VariableName=Fx_fr  SaveFormat=Timeseries  SampleTime=-1
  To Workspace2 : ToWorkspace  VariableName=Fx_rl  SaveFormat=Timeseries  SampleTime=-1
  To Workspace3 : ToWorkspace  VariableName=Fx_rr  SaveFormat=Timeseries  SampleTime=-1
  Visualise Fx tire : Scope  NumInputPorts=4
      settings: ActiveDisplayYMinimum=-1  ActiveDisplayYMaximum=1  DataLoggingVariableName=ScopeData4
  wires:
  Fx_tire/1 -> MATLAB Function/1(Fx_tire)
  MATLAB Function/1(Fx_fl) -> Visualise Fx tire/1, To Workspace/1  "Fx_fl"
  MATLAB Function/2(Fx_fr) -> Visualise Fx tire/2, To Workspace1/1  "Fx_fr"
  MATLAB Function/3(Fx_rl) -> Visualise Fx tire/3, To Workspace2/1  "Fx_rl"
  MATLAB Function/4(Fx_rr) -> Visualise Fx tire/4, To Workspace3/1  "Fx_rr"

== system vehicle_model_2025/Visualise_Fx_tire1 ==
  Fz_tire : Inport
  MATLAB Function : MATLAB Function  TreatAsAtomicUnit=on
  To Workspace : ToWorkspace  VariableName=Fz_fl  SaveFormat=Timeseries  SampleTime=-1
  To Workspace1 : ToWorkspace  VariableName=Fz_fr  SaveFormat=Timeseries  SampleTime=-1
  To Workspace2 : ToWorkspace  VariableName=Fz_rl  SaveFormat=Timeseries  SampleTime=-1
  To Workspace3 : ToWorkspace  VariableName=Fz_rr  SaveFormat=Timeseries  SampleTime=-1
  Visualise Fz tire : Scope  NumInputPorts=4
      settings: ActiveDisplayYMinimum=574.34880299507154  ActiveDisplayYMaximum=755.17925514733838  DataLoggingVariableName=ScopeData4
  wires:
  MATLAB Function/4(Fz_rr) -> To Workspace3/1, Visualise Fz tire/4  "Fz_rr"
  MATLAB Function/3(Fz_rl) -> To Workspace2/1, Visualise Fz tire/3  "Fz_rl"
  MATLAB Function/2(Fz_fr) -> To Workspace1/1, Visualise Fz tire/2  "Fz_fr"
  MATLAB Function/1(Fz_fl) -> To Workspace/1, Visualise Fz tire/1  "Fz_fl"
  Fz_tire/1 -> MATLAB Function/1(Fz_tire)

== system vehicle_model_2025/Visualise_Fy_tire ==
  Fy_tire : Inport
  MATLAB Function : MATLAB Function  TreatAsAtomicUnit=on
  To Workspace : ToWorkspace  VariableName=Fy_fl  SaveFormat=Timeseries  SampleTime=-1
  To Workspace1 : ToWorkspace  VariableName=Fy_fr  SaveFormat=Timeseries  SampleTime=-1
  To Workspace2 : ToWorkspace  VariableName=Fy_rl  SaveFormat=Timeseries  SampleTime=-1
  To Workspace3 : ToWorkspace  VariableName=Fy_rr  SaveFormat=Timeseries  SampleTime=-1
  Visualise Fy tire : Scope  NumInputPorts=4
      settings: ActiveDisplayYMinimum=-1  ActiveDisplayYMaximum=1  DataLoggingVariableName=ScopeData12
  wires:
  Fy_tire/1 -> MATLAB Function/1(Fy_tire)
  MATLAB Function/2(Fy_fr) -> Visualise Fy tire/2, To Workspace1/1  "Fy_fr"
  MATLAB Function/4(Fy_rr) -> Visualise Fy tire/4, To Workspace3/1  "Fy_rr"
  MATLAB Function/1(Fy_fl) -> Visualise Fy tire/1, To Workspace/1  "Fy_fl"
  MATLAB Function/3(Fy_rl) -> Visualise Fy tire/3, To Workspace2/1  "Fy_rl"

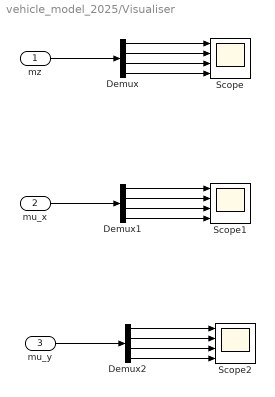
== system vehicle_model_2025/Visualiser ==
  mz : Inport
  mu_x : Inport  Port=2
  mu_y : Inport  Port=3
  Demux : Demux
  Demux1 : Demux
  Demux2 : Demux
  Scope : Scope  NumInputPorts=4
      settings: ActiveDisplayYMinimum=-1  ActiveDisplayYMaximum=1
  Scope1 : Scope  NumInputPorts=4
  Scope2 : Scope  NumInputPorts=4
  wires:
  mz/1 -> Demux/1
  Demux/1 -> Scope/1
  Demux/2 -> Scope/2
  Demux/3 -> Scope/3
  Demux/4 -> Scope/4
  Demux1/3 -> Scope1/3
  Demux1/2 -> Scope1/2
  mu_x/1 -> Demux1/1
  Demux1/1 -> Scope1/1
  Demux1/4 -> Scope1/4
  Demux2/3 -> Scope2/3
  Demux2/2 -> Scope2/2
  mu_y/1 -> Demux2/1
  Demux2/1 -> Scope2/1
  Demux2/4 -> Scope2/4

== system vehicle_model_2025/Wheel Dynamics ==
  T_in : Inport
  Fx : Inport  Port=2
  Omega : Inport  Port=3
  Fx_tire : Inport  Port=4
  Integrator : Integrator  InitialCondition=init_vx/Par.R0  LimitOutput=on  UpperSaturationLimit=1e6
  MATLAB Function : MATLAB Function  TreatAsAtomicUnit=on
  omega : Outport
  wires:
  Integrator/1 -> omega/1
  T_in/1 -> MATLAB Function/1(T_in)
  Fx/1 -> MATLAB Function/2(Fx_rr)
  Omega/1 -> MATLAB Function/4(Omega)
  MATLAB Function/1(Omega_dot) -> Integrator/1
  Fx_tire/1 -> MATLAB Function/3(Fx_tire)

== system vehicle_model_2025/roll and pitch angles ==
  ax : Inport
  ay : Inport  Port=2
  F_aero : Inport  Port=3
  Phi_constants : MATLAB Function  TreatAsAtomicUnit=on
  Pitch : Subsystem
  Roll : Subsystem
  theta_constants : MATLAB Function  TreatAsAtomicUnit=on
  phi : Outport
  Theta : Outport  Port=2
  wires:
  ax/1 -> Pitch/3(ax)
  Phi_constants/1(K_phi) -> Roll/1(K_phi)
  Phi_constants/2(C_phi) -> Roll/2(C_phi)
  ay/1 -> Roll/3(ay)
  Roll/1(phi) -> phi/1
  Pitch/1(Theta) -> Theta/1
  theta_constants/1(K_theta) -> Pitch/1(K_theta)
  theta_constants/2(C_theta) -> Pitch/2(C_theta)
  F_aero/1 -> Pitch/4(downforce)

== system vehicle_model_2025/steer_input ==
  Clock : Clock
  Ramp : simulink/Sources/Ramp  slope=-pi/40  start=6  InitialOutput=pi/10
  Ramp1 : simulink/Sources/Ramp  slope=pi/40  start=2  InitialOutput=0
  Saturation : Saturate  UpperLimit=pi/10  LowerLimit=0
  Switch : Switch  Criteria=u2 > Threshold  Threshold=6  SaturateOnIntegerOverflow=off  InputSameDT=off
  steer_input : Outport
  wires:
  Switch/1 -> Saturation/1
  Ramp/1 -> Switch/1
  Ramp1/1 -> Switch/3
  Clock/1 -> Switch/2
  Saturation/1 -> steer_input/1  "steer_input"

== system vehicle_model_2025/throttle_input ==
  Constant : Constant
  Saturation : Saturate  UpperLimit=1  LowerLimit=0
  Out1 : Outport
  wires:
  Constant/1 -> Saturation/1
  Saturation/1 -> Out1/1

== system vehicle_model_2025/visualise input ==
  InputBus : Inport
  Add : Sum
  Bus Creator : BusCreator  Inputs=4
  Bus Selector : BusSelector  OutputSignals=Torque_input,Steer_input
  Bus Selector1 : BusSelector  OutputSignals=signal3,signal4
  Demux : Demux
  Scope : Scope  NumInputPorts=2
      settings: ActiveDisplayYMinimum=-60.684412499999979  ActiveDisplayYMaximum=546.1597125  DataLoggingVariableName=ScopeData10
  Terminator : Terminator
  wires:
  InputBus/1 -> Bus Selector/1
  Bus Selector/2 -> Scope/2  "<Steer_input>"
  Bus Selector/1 -> Demux/1  "<Torque_input>"
  Demux/1 -> Bus Creator/1
  Demux/2 -> Bus Creator/2
  Demux/3 -> Bus Creator/3
  Demux/4 -> Bus Creator/4
  Bus Creator/1 -> Bus Selector1/1
  Bus Selector1/1 -> Add/2  "<signal3>"
  Bus Selector1/2 -> Add/1  "<signal4>"
  Add/1 -> Scope/1, Terminator/1  "Total_torque"

== system vehicle_model_2025/Force and Torque Equilibrium/disp=75 ==
  disp : Inport
  Clock : Clock
  Compare To Constant : simulink/Logic and Bit Operations/Compare To Constant  relop=>=  const=75  OutDataTypeStr=boolean
  Detect Rise Positive : simulink/Logic and Bit Operations/Detect Rise Positive  vinit=0  OutDataTypeStr=boolean
  Triggered Subsystem : Subsystem  TreatAsAtomicUnit=on
  Out1 : Outport
  wires:
  Detect Rise Positive/1 -> Triggered Subsystem/Trigger
  Clock/1 -> Triggered Subsystem/1(In1)
  Compare To Constant/1 -> Detect Rise Positive/1
  Triggered Subsystem/1(Out1) -> Out1/1
  disp/1 -> Compare To Constant/1

== system vehicle_model_2025/Normal_loads/ARB ==
  Zs : Inport
  MATLAB Function : MATLAB Function  TreatAsAtomicUnit=on
  Subsystem : Subsystem
  F_arb : Outport
  wires:
  Zs/1 -> MATLAB Function/1(Zs)
  MATLAB Function/1(F_arb) -> Subsystem/1(F_arb), F_arb/1

== system vehicle_model_2025/Normal_loads/Spring_forces ==
  theta : Inport
  phi : Inport  Port=2
  F_aero : Inport  Port=3
  MATLAB Function : MATLAB Function  TreatAsAtomicUnit=on
  Zs : Outport
  F_spring : Outport  Port=2
  wires:
  theta/1 -> MATLAB Function/1(theta)
  phi/1 -> MATLAB Function/2(phi)
  F_aero/1 -> MATLAB Function/3(F_aero_total)
  MATLAB Function/2(F_spring) -> F_spring/1
  MATLAB Function/1(Zs) -> Zs/1

== system vehicle_model_2025/Normal_loads/Visualise F_spring ==
  Zs : Inport
  Demux : Demux
  Gain : Gain  Gain=-1
  Scope : Scope  NumInputPorts=4
      settings: ActiveDisplayYMinimum=514.60494659064307  ActiveDisplayYMaximum=1379.8102505236993  DataLoggingVariableName=ScopeData26
  wires:
  Zs/1 -> Gain/1
  Demux/1 -> Scope/1
  Demux/2 -> Scope/2
  Demux/3 -> Scope/3
  Demux/4 -> Scope/4
  Gain/1 -> Demux/1

== system vehicle_model_2025/Normal_loads/Visualise sus disp ==
  Zs : Inport
  MATLAB Function : MATLAB Function  TreatAsAtomicUnit=on
  Scope : Scope  NumInputPorts=4
      settings: ActiveDisplayYMinimum=-0.1034097371737408  ActiveDisplayYMaximum=0.016260925393945278  DataLoggingVariableName=ScopeData26
  wires:
  Zs/1 -> MATLAB Function/1(Zs)
  MATLAB Function/1(zsfl) -> Scope/1
  MATLAB Function/2(zsfr) -> Scope/2
  MATLAB Function/3(zsrl) -> Scope/3
  MATLAB Function/4(zsrr) -> Scope/4

== system vehicle_model_2025/Normal_loads/Visualise sus disp1 ==
  F_z : Inport
  Demux : Demux
  Scope : Scope  NumInputPorts=4
      settings: ActiveDisplayYMinimum=500.38210116997504  ActiveDisplayYMaximum=1507.8158593097112  DataLoggingVariableName=ScopeData26
  wires:
  Demux/4 -> Scope/4
  Demux/3 -> Scope/3
  Demux/2 -> Scope/2
  Demux/1 -> Scope/1
  F_z/1 -> Demux/1

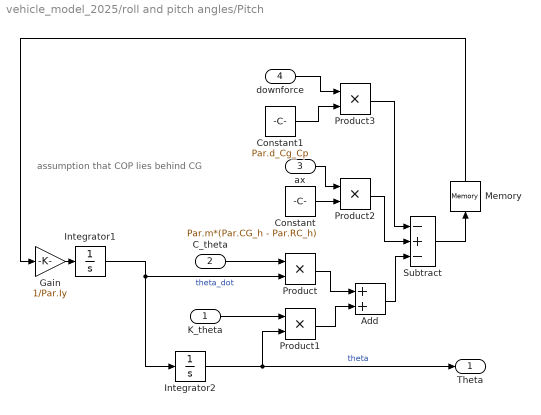
== system vehicle_model_2025/roll and pitch angles/Pitch ==
  note: assumption that COP lies behind CG
  K_theta : Inport
  C_theta : Inport  Port=2
  ax : Inport  Port=3
  downforce : Inport  Port=4
  Add : Sum
  Constant : Constant  Value=Par.m*(Par.CG_h - Par.RC_h)
  Constant1 : Constant  Value=Par.d_Cg_Cp
  Gain : Gain  Gain=1/Par.Iy
  Integrator1 : Integrator
  Integrator2 : Integrator
  Memory : Memory
  Product{,1..3} (4 alike) : Product
  Subtract : Sum  Inputs=-+-
  Theta : Outport
  wires:
  Gain/1 -> Integrator1/1
  Integrator1/1 -> Product/2, Integrator2/1  "theta_dot"
  C_theta/1 -> Product/1
  Integrator2/1 -> Theta/1, Product1/2  "theta"
  K_theta/1 -> Product1/1
  Product/1 -> Add/1
  Product1/1 -> Add/2
  ax/1 -> Product2/1
  Constant/1 -> Product2/2
  Product2/1 -> Subtract/2
  Add/1 -> Subtract/3
  Subtract/1 -> Memory/1
  Memory/1 -> Gain/1
  downforce/1 -> Product3/1
  Constant1/1 -> Product3/2
  Product3/1 -> Subtract/1

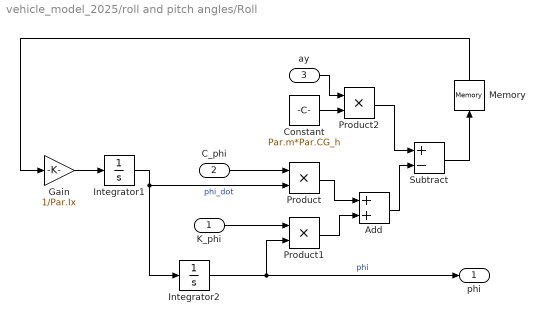
== system vehicle_model_2025/roll and pitch angles/Roll ==
  K_phi : Inport
  C_phi : Inport  Port=2
  ay : Inport  Port=3
  Add : Sum
  Constant : Constant  Value=Par.m*Par.CG_h
  Gain : Gain  Gain=1/Par.Ix
  Integrator1 : Integrator
  Integrator2 : Integrator
  Memory : Memory
  Product : Product
  Product1 : Product
  Product2 : Product
  Subtract : Sum  Inputs=+-
  phi : Outport
  wires:
  Subtract/1 -> Memory/1
  Add/1 -> Subtract/2
  Product2/1 -> Subtract/1
  Constant/1 -> Product2/2
  ay/1 -> Product2/1
  Product1/1 -> Add/2
  Product/1 -> Add/1
  K_phi/1 -> Product1/1
  Integrator2/1 -> Product1/2, phi/1  "phi"
  C_phi/1 -> Product/1
  Integrator1/1 -> Integrator2/1, Product/2  "phi_dot"
  Gain/1 -> Integrator1/1
  Memory/1 -> Gain/1

== system vehicle_model_2025/Force and Torque Equilibrium/disp=75/Triggered Subsystem ==
  In1 : Inport
  Trigger : TriggerPort  VariantControl=(inherit)
  Out1 : Outport
  wires:
  In1/1 -> Out1/1

== system vehicle_model_2025/Normal_loads/ARB/Subsystem ==
  F_arb : Inport
  Demux : Demux
  Scope : Scope  NumInputPorts=4
      settings: ActiveDisplayYMinimum=-1  ActiveDisplayYMaximum=1  DataLoggingVariableName=ScopeData11
  wires:
  F_arb/1 -> Demux/1
  Demux/1 -> Scope/1  "F_arb_fl"
  Demux/2 -> Scope/2  "F_arb_fr"
  Demux/3 -> Scope/3  "F_arb_rl"
  Demux/4 -> Scope/4  "F_arb_rr"

== matlab function vehicle_model_2025/Rolling and Drag forces/Rolling Forces ==
  data: Fz input; Fx_rr_b output; Steer_FL input; Steer_FR input; Fy_rr_b output; Par parameter
function [Fx_rr_b, Fy_rr_b] = fcn(Fz, Steer_FL, Steer_FR, Par)

    %#codegen

    % 1. Setup
    C_rr = Par.C_rr; 
    
    % Construct Steering Vector (Assuming Rear Steer = 0)
    Delta = [Steer_FL; Steer_FR; 0; 0];

    % Initialize Outputs
    Fx_rr_b = zeros(4, 1);
    Fy_rr_b = zeros(4, 1);

    % 2. Calculate & Resolve Forces (Vectorized Loop)
    for i = 1:4
        
        % Magnitude (Always positive Fz)
        F_mag = C_rr * abs(Fz(i));
        
        % B. Define Force Vector in Wheel Frame
        F_xw = -F_mag;
        F_yw = 0;
        
        % C. Transform to Body Frame (Rotation)
        d = Delta(i);
        c = cos(d);
        s = sin(d);
        
        % Rotate: F_body = Rz(delta) * F_wheel
        % Fx_b = Fx_w*cos - Fy_w*sin
        Fx_rr_b(i) = F_xw * c - F_yw * s;
        
        % Fy_b = Fx_w*sin + Fy_w*cos
        Fy_rr_b(i) = F_xw * s + F_yw * c;
    end

end

== matlab function vehicle_model_2025/Force and Torque Equilibrium/Force and Torque Equilibrium ==
  data: B_Fx input; ax output size=1; ay output size=1; B_Fy input; B_Fx_roll input; B_Fy_roll input; B_F_drag input; yawrate input; vx input; vy input; yawmoment output size=1; Par parameter
function [ax, ay, yawmoment] = fcn(B_Fx, B_Fy, B_Fx_roll, B_Fy_roll, B_F_drag, yawrate, vx, vy, Par)
%#codegen

    % 1. Geometry Setup
    m = Par.m;
    Iz = Par.Iz;
    a = Par.Lf;     % CG to Front Axle
    b = Par.Lr;     % CG to Rear Axle
    half_T = Par.TW / 2; 

    % 2. Combine Forces at Each Corner (Traction + Rolling)

    Fx_total = B_Fx + B_Fx_roll; 
    Fy_total = B_Fy + B_Fy_roll; 
    
    % 3. Force Equilibrium
    Sigma_Fx = sum(Fx_total) - B_F_drag(1);
    Sigma_Fy = sum(Fy_total) ;
    
    % 4. Linear Accelerations 

    ax = (Sigma_Fx / m) + (vy * yawrate);
    ay = (Sigma_Fy / m) - (vx * yawrate);
    
    % --- Front Left (Index 1) ---
    % x = +a, y = +half_T
    M_FL = (a * Fy_total(1)) - (half_T * Fx_total(1));
    
    % --- Front Right (Index 2) ---
    % x = +a, y = -half_T
    % Note: -(-half_T) becomes +half_T
    M_FR = (a * Fy_total(2)) - (-half_T * Fx_total(2));
    
    % --- Rear Left (Index 3) ---
    % x = -b, y = +half_T
    M_RL = (-b * Fy_total(3)) - (half_T * Fx_total(3));
    
    % --- Rear Right (Index 4) ---
    % x = -b, y = -half_T
    M_RR = (-b * Fy_total(4)) - (-half_T * Fx_total(4));
    
    % 6. Total Yaw Moment & Acceleration
    Sigma_Mz = M_FL + M_FR + M_RL + M_RR;
    yawmoment = Sigma_Mz / Iz;

end

== matlab function vehicle_model_2025/Rolling and Drag forces/Aero Drag ==
  data: vx input; B_F_aero output; vy input; aero_par parameter
function B_F_aero = fcn(vx, vy, aero_par)

    %#codegen
    % AERODYNAMIC DRAG (Body Frame)
    % Calculates drag vector acting on the CG.
%
% Inputs:
%   vx, vy : Vehicle Velocities in Body Frame [m/s]
%   Par    : Parameters (.Cd, .Area, .rho, .C_side)
%
% Output:
%   B_F_aero : [Fx; Fy; 0] Aerodynamic Force Vector [N]

    % 1. Longitudinal Drag (Standard)
    % Fx = -0.5 * rho * Cd * Area * vx^2
    % Usage: sign(vx) ensures drag always opposes motion
    Fx_drag = 0.5 * aero_par.rho * aero_par.Cd * aero_par.Area * vx * abs(vx);

    % 2. Lateral Drag (Side Force) - Optional
    % Only relevant if sliding significantly.
    % If Par.C_side is not defined, calculate as 0.
    if isfield(aero_par, 'C_side') && aero_par.C_side > 0
        % Side area is often approx same as Frontal Area or larger
        % Fy = -0.5 * rho * C_side * Area_Side * vy^2
        Fy_drag = -0.5 * aero_par.rho * aero_par.C_side * aero_par.Area * vy * abs(vy);
    else
        Fy_drag = 0;
    end
    
    % 3. Output Vector for Equilibrium Block
    B_F_aero = [Fx_drag; Fy_drag; 0];

end

== matlab function vehicle_model_2025/Toe_including_compliances/toe_fl ==
  data: Fy_tire input; Fx_tire input; Toe output; Mz input; sus_par parameter
function Toe = fcn(Fy_tire,Fx_tire,Mz,sus_par)

Toe= sus_par.Toe_f_static + sus_par.C_Fx_toe.*Fx_tire + sus_par.C_Fy_toe.*Fy_tire + sus_par.C_Mz_toe.*Mz;

== matlab function vehicle_model_2025/Toe_including_compliances/toe_fr ==
  data: Toe output; Mz input; Fx_tire input; Fy_tire input; sus_par parameter
function Toe = fcn(Mz,Fx_tire,Fy_tire,sus_par)

Toe= sus_par.Toe_f_static + sus_par.C_Fx_toe.*Fx_tire + sus_par.C_Fy_toe.*Fy_tire + sus_par.C_Mz_toe.*Mz;

== matlab function vehicle_model_2025/Toe_including_compliances/toe_rl ==
  data: Fy_tire input; Fx_tire input; Toe output; Mz input; sus_par parameter
function Toe = fcn(Fy_tire,Fx_tire,Mz,sus_par)

Toe = sus_par.Toe_r_static + sus_par.C_Fx_toe.*Fx_tire + sus_par.C_Fy_toe.*Fy_tire + sus_par.C_Mz_toe.*Mz;

== matlab function vehicle_model_2025/Toe_including_compliances/toe_rr ==
  data: Toe output; Mz input; Fx_tire input; Fy_tire input; sus_par parameter
function Toe = fcn(Mz,Fx_tire,Fy_tire,sus_par)

Toe = sus_par.Toe_r_static + sus_par.C_Fx_toe.*Fx_tire + sus_par.C_Fy_toe.*Fy_tire + sus_par.C_Mz_toe.*Mz;
